simulink model "uz_FOC"  (R2021a)
settings: Solver=FixedStepDiscrete  StartTime=0.0  StopTime=50.0  FixedStep=0.00001  RelTol=1e-3  EnableMultiTasking=on
values from neighbouring files (symbols this model uses):
  d_d_TMS = 0.005    [uz_FOC_init.m]
  d_f_c = 100000    [uz_FOC_init.m]
  d_i_max = 15    [uz_FOC_init.m]
  d_i_min = -d_i_max    (= -15)    [uz_FOC_init.m]
  d_J_Coupling_M_E = 2e-6    (= 2e-06)    [uz_FOC_init.m]
  d_J_Coupling_M_Ms = 2e-20    [uz_FOC_init.m]
  d_J_Ms_L = d_J_Ms_M    (= 1.26363648e-05)    [uz_FOC_init.m]
  d_J_Ms_M = 0.5*0.5*((0.5*d_d_Ms)^4)*3.14*d_l_Ms*d_rho_Ms    (= 1.26363648e-05)    [uz_FOC_init.m]
  d_Ki_id = d_Kp_id/d_Tn_id    (= 125)    [uz_FOC_init.m]
  d_Ki_iq = d_Kp_iq/d_Tn_iq    (= 125)    [uz_FOC_init.m]
  d_Ki_n = d_Kp_n/d_Tn_n    (= 0.003888)    [uz_FOC_init.m]
  d_Kp_id = d_L_d / (4*20/d_f_c)    (= 0.25)    [uz_FOC_init.m]
  d_Kp_iq = d_L_q / (4*20/d_f_c)    (= 0.375)    [uz_FOC_init.m]
  d_Kp_n = 0.00864*0.045    (= 0.0003888)    [uz_FOC_init.m]
  d_L_d = 0.0002    [uz_FOC_init.m]
  d_L_q = 0.0003    [uz_FOC_init.m]
  d_p = 4    [uz_FOC_init.m]
  d_psi_pm = 0.0075    [uz_FOC_init.m]
  d_R_ph = d_R_ph_ph/2    (= 0.1)    [uz_FOC_init.m]
  d_y_max = 10    [uz_FOC_init.m]
  d_y_min = -d_y_max    (= -10)    [uz_FOC_init.m]
undefined symbols (not defined in the file or in its folder): i_d, i_q, para, u_d, u_q
libraries: fl_lib x44, nesl_utility x27, ee_lib x21, simulink x8, spsabctodq0Lib x2, spsTriangleGeneratorLib x1, eeTransforms x1
(part 1 of 3)
settings Model: PacingRate=0.010000  Creator=Hufnagel  LastModifiedBy=hufnagelde
settings SolverCC: AutoInsertRateTranBlk=on
settings DataIOCC: SaveOutput=off  SignalLogging=off  DSMLogging=off  SaveTime=off
settings OptimizationCC: DefaultParameterBehavior=Inlined  UseDivisionForNetSlopeComputation=on  GainParamInheritBuiltInType=on  UseFloatMulNetSlope=on  DefaultUnderspecifiedDataType=single  EnhancedBackFolding=on  PassReuseOutputArgsAs=Individual arguments  OptimizeBlockOrder=speed  DifferentSizesBufferReuse=on  OptimizationCustomize=off  EfficientTunableParamExpr=on
settings DebuggingCC: ParameterTunabilityLossMsg=error
settings SFSimCC: MATLABDynamicMemAlloc=off
settings RTWCC: SystemTargetFile=ert.tlc  GenCodeOnly=on  TemplateMakefile=ert_default_tmf  GenerateReport=on  BuildConfiguration=Faster Runs  GenerateCodeMetricsReport=on  CheckMdlBeforeBuild=Warning
settings CodeAppCC: ForceParamTrailComments=on  IgnoreCustomStorageClasses=off  OperatorAnnotations=on  SimulinkDataObjDesc=on  SFDataObjDesc=on  CustomSymbolStrGlobalVar=rt$N$M  CustomSymbolStrType=$N$M  CustomSymbolStrFcn=$N$M$F  CustomSymbolStrMacro=$N$M  InsertBlockDesc=on
settings ERTTargetCC: TargetLangStandard=C99 (ISO)  SuppressErrorStatus=on  IncludeFileDelimiter=UseQuote  SupportAbsoluteTime=off  CodeInterfacePackaging=Reusable function  SupportNonFinite=off  InlinedParameterPlacement=NonHierarchical  MultiInstanceErrorCode=Warning  RootIOFormat=Part of model data structure  ERTCustomFileTemplate=example_file_process.tlc  GlobalDataDefinition=InSourceFile  GlobalDataReference=InSourceFile  ERTFilePackagingFormat=CompactWithDataFile

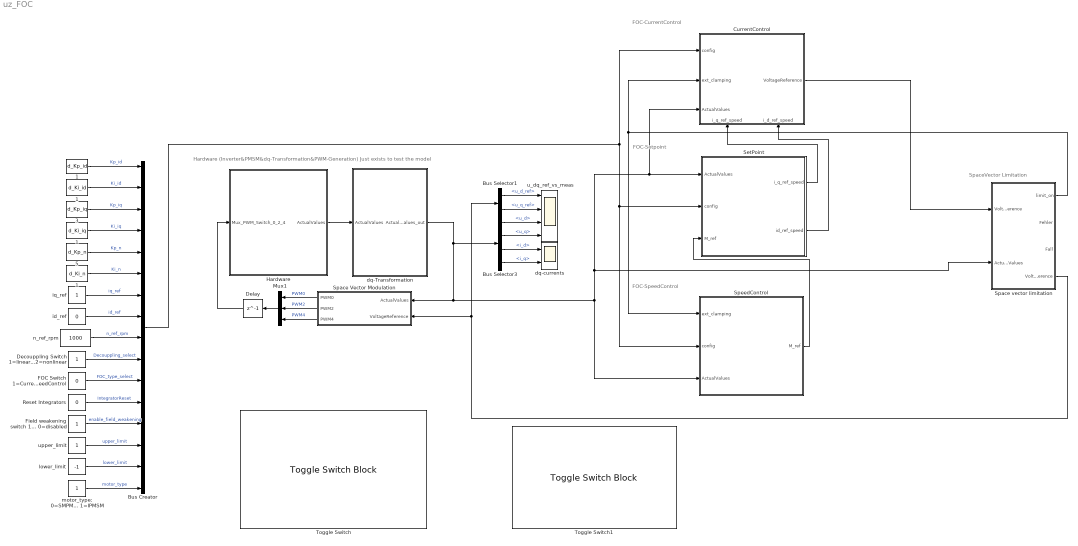
== system uz_FOC ==
  note: SpaceVector Limitation
  note: FOC-SpeedControl
  note: FOC-CurrentControl
  note: Hardware (Inverter&PMSM&dq-Transformation&PWM-Generation)
      | Just exists to test the model
  note: FOC-Setpoint
  "         1" : Constant  Value=d_Ki_n  OutDataTypeStr=single  SampleTime=1/d_f_c
  "       1" : Constant  Value=d_Ki_id  OutDataTypeStr=single  SampleTime=1/d_f_c
  "    1" : Constant  Value=d_Ki_iq  OutDataTypeStr=single  SampleTime=1/d_f_c
  "  1" : Constant  Value=d_Kp_id  OutDataTypeStr=single  SampleTime=1/d_f_c
  "  3" : Constant  Value=d_Kp_iq  OutDataTypeStr=single  SampleTime=1/d_f_c
  "  5" : Constant  Value=d_Kp_n  OutDataTypeStr=single  SampleTime=1/d_f_c
  Bus Creator : BusCreator  Inputs=16  OutDataTypeStr=Bus: config
  Bus Selector1 : BusSelector  OutputSignals=u_d_ref,u_q_ref
  Bus Selector3 : BusSelector  OutputSignals=u_d,u_q,i_d,i_q
  CurrentControl : Subsystem
      settings: PortSchema="{\"entries\":[{\"content\":{\"sides\":[{\"content\":{\"connectorIds\":[\"In1\",\"In2\",\"In3\"]},\"type\":\"ConnectorPlacement.EquallySpacedRectSide\",\"uuid\":\"77c09fd7-fff9-4bf9-9e3c-ae7d8d4ae844\"},{\"content\":{\"connectorIds\":[\"Out1\"],\"side\":\"RIGHT\"},\"type\":\"ConnectorPlacement.EquallySpacedRectSide\",\"uuid\":\"d9a85257-d7d2-47a7-af12-4b0d4d0582bd\"},{\"content\":{\"connectorIds\":[],\"side\":\"TOP\"},\"type\":\"ConnectorPlacement.EquallySpacedRectSide\",\"uuid\":\"c30896ce-cf5a-4a2d-9d70-70e47f59ac53\"},{\"content\":{\"connectorIds\":[\"In4\",\"In5\"],\"side\":\"BOTTOM\"},\"type\":\"ConnectorPlacement.EquallySpacedRectSide\",\"uuid\":\"4956357e-f10e-445a-971a-b0f87868dbb6\"}]},\"type\":\"ConnectorPlacement.EquallySpacedConnector\",\"uuid\":\"e52ebb7a-573d-4053-a7f6-74acae9243d3\"}],\"packageUris\":[\"http://schema.mathworks.com/mf0/Connector/R2020b\"],\"version\":\"1.0\"}"
  Decouppling Switch 1=linear 2=nonlinear : Constant  OutDataTypeStr=boolean
  Delay : Delay  DelayLength=1  InitialCondition=0
  FOC Switch 1=CurrentControl 0=SpeedControl : Constant  Value=0  OutDataTypeStr=boolean
  Field weakening switch 1=enabled 0=disabled : Constant  OutDataTypeStr=boolean
  Hardware : Subsystem
  Mux1 : Mux  Inputs=3
  Reset Integrators : Constant  Value=0  OutDataTypeStr=boolean  SampleTime=1/d_f_c
  SetPoint : Subsystem
  Space Vector Modulation : Subsystem
  Space vector limitation : MATLAB Function  TreatAsAtomicUnit=on
  SpeedControl : Subsystem
  Toggle Switch : ToggleSwitchBlock
      settings: Values={{'SpeedControl', 'CurrentControl'}, [0 1]}
  Toggle Switch1 : ToggleSwitchBlock
      settings: Values={{'Nonlinear Decouppling', 'Linear Decouppling'}, [0 1]}
  dq-Transformation : Subsystem
  dq-currents : Scope  NumInputPorts=2
  id_ref : Constant  Value=0  OutDataTypeStr=single
  iq_ref : Constant  OutDataTypeStr=single
  lower_limit : Constant  Value=-1  OutDataTypeStr=single
  motor_type: 0=SMPMSM 1=IPMSM : Constant  OutDataTypeStr=uint16
  n_ref_rpm : Constant  Value=1000  OutDataTypeStr=single  SampleTime=1/d_f_c
  u_dq_ref_vs_meas : Scope  NumInputPorts=4
  upper_limit : Constant  OutDataTypeStr=single
  wires:
  Space Vector Modulation/1(PWM0) -> Mux1/1  "PWM0"
  Space Vector Modulation/2(PWM2) -> Mux1/2  "PWM2"
  Space Vector Modulation/3(PWM4) -> Mux1/3  "PWM4"
  Mux1/1 -> Delay/1
  Delay/1 -> Hardware/1(Mux_PWM_Switch_0_2_4)
  "  1"/1 -> Bus Creator/1  "Kp_id"
  "       1"/1 -> Bus Creator/2  "Ki_id"
  "  3"/1 -> Bus Creator/3  "Kp_iq"
  "    1"/1 -> Bus Creator/4  "Ki_iq"
  "  5"/1 -> Bus Creator/5  "Kp_n"
  "         1"/1 -> Bus Creator/6  "Ki_n"
  iq_ref/1 -> Bus Creator/7  "iq_ref"
  id_ref/1 -> Bus Creator/8  "id_ref"
  Decouppling Switch 1=linear 2=nonlinear/1 -> Bus Creator/10  "Decouppling_select"
  Hardware/1(ActualValues) -> dq-Transformation/1(ActualValues)
  dq-Transformation/1(ActualValues_out) -> CurrentControl/3(ActualValues), SetPoint/1(ActualValues), Space vector limitation/2(ActualValues), SpeedControl/3(ActualValues), Space Vector Modulation/1(ActualValues), Bus Selector3/1
  CurrentControl/1(VoltageReference) -> Space vector limitation/1("VoltageReference ")
  FOC Switch 1=CurrentControl 0=SpeedControl/1 -> Bus Creator/11  "FOC_type_select"
  Bus Selector3/2 -> u_dq_ref_vs_meas/4  "<u_q>"
  Bus Selector3/1 -> u_dq_ref_vs_meas/3  "<u_d>"
  Bus Selector3/3 -> dq-currents/1  "<i_d>"
  Bus Selector3/4 -> dq-currents/2  "<i_q>"
  Space vector limitation/4(VoltageReference) -> Bus Selector1/1, Space Vector Modulation/2(VoltageReference)
  Bus Selector1/1 -> u_dq_ref_vs_meas/1  "<u_d_ref>"
  Bus Selector1/2 -> u_dq_ref_vs_meas/2  "<u_q_ref>"
  Reset Integrators/1 -> Bus Creator/12  "IntegratorReset"
  Field weakening switch 1=enabled 0=disabled/1 -> Bus Creator/13  "enable_field_weakening"
  lower_limit/1 -> Bus Creator/15  "lower_limit"
  upper_limit/1 -> Bus Creator/14  "upper_limit"
  SpeedControl/1(M_ref) -> SetPoint/3(M_ref)
  SetPoint/1(i_q_ref_speed) -> CurrentControl/4(i_q_ref_speed)
  SetPoint/2(id_ref_speed) -> CurrentControl/5(i_d_ref_speed)
  Space vector limitation/1(limit_on) -> SpeedControl/1(ext_clamping), CurrentControl/2(ext_clamping)
  Bus Creator/1 -> CurrentControl/1(config), SpeedControl/2(config), SetPoint/2(config)
  motor_type: 0=SMPMSM 1=IPMSM/1 -> Bus Creator/16  "motor_type"
  n_ref_rpm/1 -> Bus Creator/9  "n_ref_rpm"

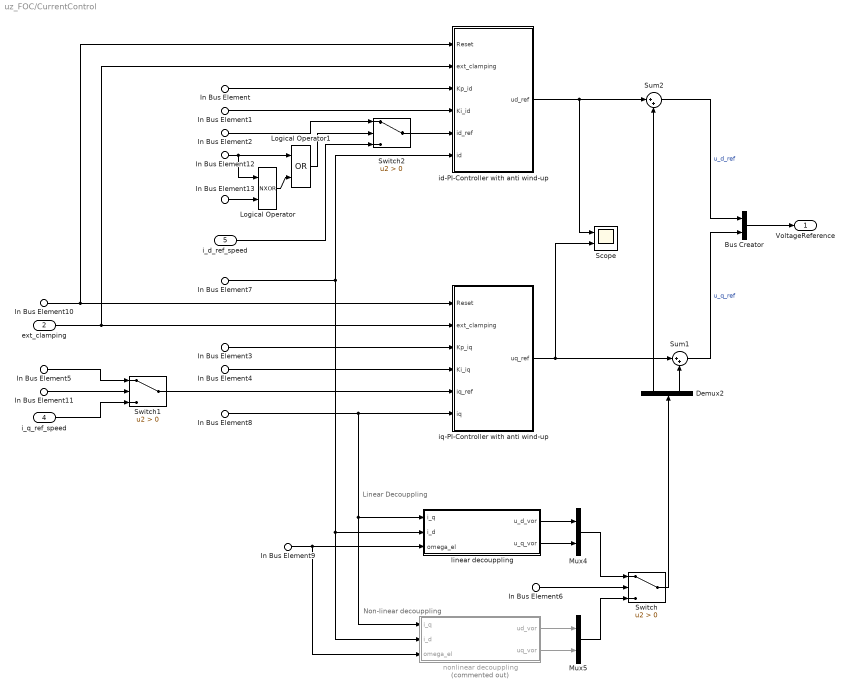
== system uz_FOC/CurrentControl ==
  note: Linear Decouppling
  note: Non-linear decouppling
  In Bus Element : Inport  PortName=config  Element=Kp_id
  In Bus Element1 : Inport  PortName=config  Element=Ki_id
  In Bus Element3 : Inport  PortName=config  Element=Kp_iq
  In Bus Element4 : Inport  PortName=config  Element=Ki_iq
  In Bus Element5 : Inport  PortName=config  Element=iq_ref
  In Bus Element6 : Inport  PortName=config  Element=Decouppling_select
  In Bus Element11 : Inport  PortName=config  Element=FOC_type_select
  In Bus Element12 : Inport  PortName=config  Element=FOC_type_select
  In Bus Element10 : Inport  PortName=config  Element=IntegratorReset
  In Bus Element2 : Inport  PortName=config  Element=id_ref
  In Bus Element13 : Inport  PortName=config  Element=enable_field_weakening
  ext_clamping : Inport  Port=2
  In Bus Element9 : Inport  Port=3  PortName=ActualValues  Element=omega_el
  In Bus Element7 : Inport  Port=3  PortName=ActualValues  Element=i_d
  In Bus Element8 : Inport  Port=3  PortName=ActualValues  Element=i_q
  i_q_ref_speed : Inport  Port=4
  i_d_ref_speed : Inport  Port=5
  Bus Creator : BusCreator  Inputs=2  OutDataTypeStr=Bus: VoltageReference
  Demux2 : Demux  Outputs=2
  Logical Operator : Logic  Operator=NXOR  AllPortsSameDT=off  OutDataTypeStr=boolean
  Logical Operator1 : Logic  Operator=OR  AllPortsSameDT=off  OutDataTypeStr=boolean
  Mux4 : Mux  Inputs=2
  Mux5 : Mux  Inputs=2
  Scope : Scope  NumInputPorts=2
  Sum1 : Sum  Inputs=|++
  Sum2 : Sum  Inputs=|++
  Switch : Switch  Criteria=u2 > Threshold
  Switch1 : Switch  Criteria=u2 > Threshold
  Switch2 : Switch  Criteria=u2 > Threshold
  id-PI-Controller with anti wind-up : Subsystem
  iq-PI-Controller with anti wind-up : Subsystem
  linear decouppling : Subsystem
  nonlinear decouppling : Subsystem  Commented=on
  VoltageReference : Outport  OutDataTypeStr=Bus: VoltageReference
  wires:
  In Bus Element7/1 -> id-PI-Controller with anti wind-up/6(id), nonlinear decouppling/2(i_d), linear decouppling/2(i_d)
  In Bus Element1/1 -> id-PI-Controller with anti wind-up/4(Ki_id)
  In Bus Element8/1 -> nonlinear decouppling/1(i_q), linear decouppling/1(i_q), iq-PI-Controller with anti wind-up/6(iq)
  In Bus Element4/1 -> iq-PI-Controller with anti wind-up/4(Ki_iq)
  In Bus Element/1 -> id-PI-Controller with anti wind-up/3(Kp_id)
  In Bus Element3/1 -> iq-PI-Controller with anti wind-up/3(Kp_iq)
  In Bus Element10/1 -> iq-PI-Controller with anti wind-up/1(Reset), id-PI-Controller with anti wind-up/1(Reset)
  Switch1/1 -> iq-PI-Controller with anti wind-up/5(iq_ref)
  ext_clamping/1 -> iq-PI-Controller with anti wind-up/2(ext_clamping), id-PI-Controller with anti wind-up/2(ext_clamping)
  In Bus Element9/1 -> nonlinear decouppling/3(omega_el), linear decouppling/3(omega_el)
  Mux5/1 -> Switch/3
  nonlinear decouppling/1(ud_vor) -> Mux5/1
  nonlinear decouppling/2(uq_vor) -> Mux5/2
  Mux4/1 -> Switch/1
  Switch/1 -> Demux2/1
  linear decouppling/1(u_d_vor) -> Mux4/1
  linear decouppling/2(u_q_vor) -> Mux4/2
  In Bus Element6/1 -> Switch/2
  Demux2/2 -> Sum1/2
  iq-PI-Controller with anti wind-up/1(uq_ref) -> Scope/2, Sum1/1
  id-PI-Controller with anti wind-up/1(ud_ref) -> Scope/1, Sum2/1
  Demux2/1 -> Sum2/2
  Sum1/1 -> Bus Creator/2  "u_q_ref"
  Bus Creator/1 -> VoltageReference/1
  In Bus Element5/1 -> Switch1/1
  In Bus Element11/1 -> Switch1/2
  i_q_ref_speed/1 -> Switch1/3
  Sum2/1 -> Bus Creator/1  "u_d_ref"
  In Bus Element2/1 -> Switch2/1
  i_d_ref_speed/1 -> Switch2/3
  Switch2/1 -> id-PI-Controller with anti wind-up/5(id_ref)
  In Bus Element13/1 -> Logical Operator/2
  Logical Operator1/1 -> Switch2/2
  In Bus Element12/1 -> Logical Operator/1, Logical Operator1/1
  Logical Operator/1 -> Logical Operator1/2
